simulink model "F4PhantomModelV3"  (R2023b)
settings: Solver=VariableStepAuto  StartTime=0.0  StopTime=10.0  RelTol=1e-3
values from neighbouring files (symbols this model uses):
  FTx = 0    [F4ModelCode.m]    (also in F4ModelCodeV2.m; F4ModelCodeV2Q2PartD.m)
  fTx = 0    [F4ModelCode.m]    (also in F4ModelCodeV2.m; F4ModelCodeV2Q2PartD.m)
  FTy = 0    [F4ModelCode.m]    (also in F4ModelCodeV2.m; F4ModelCodeV2Q2PartD.m)
  fTy = 0    [F4ModelCode.m]    (also in F4ModelCodeV2.m; F4ModelCodeV2Q2PartD.m)
  FTz = 0    [F4ModelCode.m]    (also in F4ModelCodeV2.m; F4ModelCodeV2Q2PartD.m)
  fTz = 0    [F4ModelCode.m]    (also in F4ModelCodeV2.m; F4ModelCodeV2Q2PartD.m)
  g = -32.2    [F4ModelCode.m]    (also in F4ModelCodeV2.m; F4ModelCodeV2Q2PartD.m; F4PhantomModelCode.m)
  Hw3Coeffs = [c_L_alpha c_L_delta_E c_L_i_H c_m_alpha c_m_delta_E c_m_i_H c_L_alphadot c_L_q c_m_alphadot c_m_q c_D_alpha]    [F4ModelCode.m]    (also in F4ModelCodeV2.m; F4ModelCodeV2Q2PartD.m; F4PhantomModelCode.m = [c_L_alpha c_L_delta_E c_L_i_H c_m_alpha c_m_delta_E c_m_i_H)
  Hw4Coeffs = [c_Y_beta c_Y_delta_A c_Y_delta_R c_n_beta c_n_delta_A c_n_delta_R c_l_beta c_l_delta_A c_l_delta_R c_l_p c_Y_p c_n_p c_l_r c_Y_r c_n_r]    [F4ModelCode.m]    (also in F4ModelCodeV2.m; F4ModelCodeV2Q2PartD.m; F4PhantomModelCode.m)
  InitialInputs = [qbar1 S_ft2 c_D_1 c_L_1 cbar_ft c_m_1 uv b_ft alphadot]    [F4ModelCode.m]    (also in F4ModelCodeV2.m; F4ModelCodeV2Q2PartD.m)
  LT = 0    [F4ModelCode.m]    (also in F4ModelCodeV2Q2PartD.m)
  lT = 0    [F4ModelCode.m]    (also in F4ModelCodeV2Q2PartD.m)
  mass = Weight/32.2    (= 1211.18012422)    [F4ModelCode.m]    (also in F4ModelCodeV2.m; F4ModelCodeV2Q2PartD.m; F4PhantomModelCode.m = 1212.157)
  MT = 0    [F4ModelCode.m]    (also in F4ModelCodeV2Q2PartD.m)
  mT = 0    [F4ModelCode.m]    (also in F4ModelCodeV2Q2PartD.m)
  NT = 0    [F4ModelCode.m]    (also in F4ModelCodeV2Q2PartD.m)
  nT = 0    [F4ModelCode.m]    (also in F4ModelCodeV2Q2PartD.m)
  P1 = 0    [F4ModelCode.m]    (also in F4ModelCodeV2.m; F4ModelCodeV2Q2PartD.m; F4PhantomModelCode.m)
  q0 = angle2quat(phidot,thetadot,psidot)    [F4ModelCode.m]    (also in F4ModelCodeV2.m; F4ModelCodeV2Q2PartD.m)
  U1 = V_P_1 * cos(alpha_rad)    [F4ModelCode.m]    (also in F4ModelCodeV2.m; F4ModelCodeV2Q2PartD.m)
  uCoeffs = [c_L_u c_D_u c_m_u]    [F4ModelCode.m]    (also in F4ModelCodeV2.m; F4ModelCodeV2Q2PartD.m; F4PhantomModelCode.m = [c_L_u c_D_u])
  uk = [c_D_delta_E c_D_q c_D_i_H c_Y_1 c_Y_betadot c_l_betadot c_n_1 c_n_betadot]    [F4ModelCode.m]    (also in F4ModelCodeV2.m; F4ModelCodeV2Q2PartD.m)
  V_P_1 = 875.6    [F4ModelCode.m]    (also in F4ModelCodeV2.m; F4ModelCodeV2Q2PartD.m; F4PhantomModelCode.m = 0)
  W1 = V_P_1 * sin(alpha_rad)    [F4ModelCode.m]    (also in F4ModelCodeV2.m; F4ModelCodeV2Q2PartD.m)
undefined symbols (not defined in the file or in its folder): THETA1
settings Model: Creator=Owner  LastModifiedBy=Owner

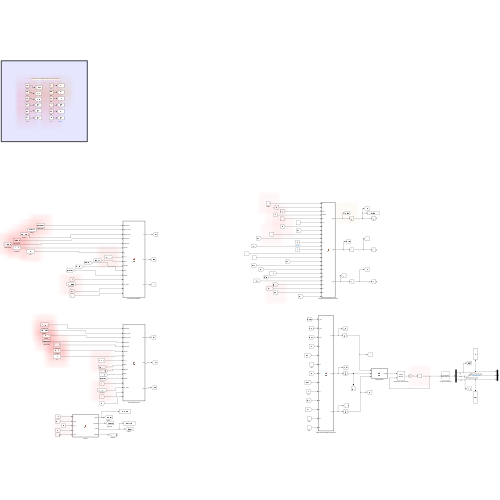
[thumbnail: Simulink's stored preview of the top-level diagram]
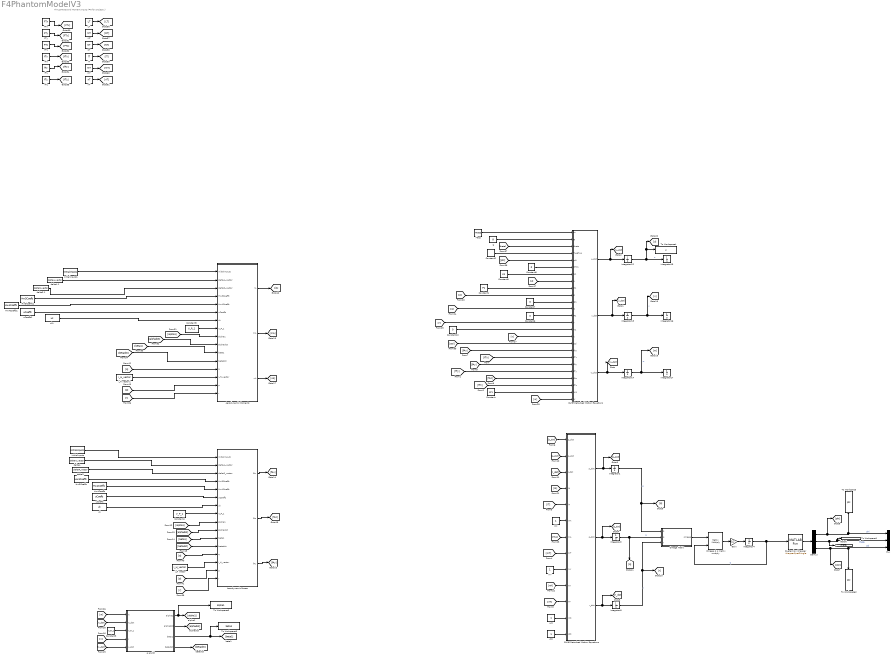
== system F4PhantomModelV3 ==
  note: Thrust Force and Moment Inputs (=0 for project 1)
  Aerodynamic Forces : MATLAB Function  TreatAsAtomicUnit=on
  Aerodynamic Moments : MATLAB Function  TreatAsAtomicUnit=on
  CAME Perturbed Motion Equations : MATLAB Function  TreatAsAtomicUnit=on
  CLME Perturbed Motion Equations : MATLAB Function  TreatAsAtomicUnit=on
  Constant : Constant  Value=W1
  Constant1 : Constant  Value=P1
  Constant{6..8,10} (4 alike) : Constant  Value=0
  Constant2 : Constant  Value=THETA1
  Constant3 : Constant  Value=V_P_1
  Constant4 : Constant  Value=V_P_1
  Constant5 : Constant  Value=V_P_1
  Constant9 : Constant  Value=U1
  Demux : Demux  Outputs=3
  FTx : Constant  Value=FTx
  FTy : Constant  Value=FTy
  FTz : Constant  Value=FTz
  Gain : Gain  Gain=1/2
  Hw3Coeffs : Constant  Value=Hw3Coeffs
  Hw3Coeffs1 : Constant  Value=Hw3Coeffs
  Hw4Coeffs : Constant  Value=Hw4Coeffs
  Hw4Coeffs1 : Constant  Value=Hw4Coeffs
  "IXX " : Constant
  IXZ : Constant
  IYY : Constant
  IZZ : Constant
  InitialInputs : Constant  Value=InitialInputs
  InitialInputs1 : Constant  Value=InitialInputs
  Integrator{1..3,12..17} (9 alike) : Integrator
  Integrator4 : Integrator  InitialCondition=q0
  LT : Constant  Value=LT
  MT : Constant  Value=MT
  Mass : Constant  Value=mass
  Mux : Mux  Inputs=3
  NT : Constant  Value=NT
  Omega & q matrix mutiply : Product  Multiplication=Matrix(*)
  Omega Matrix : MATLAB Function  TreatAsAtomicUnit=on
  Quaternion Wrapper : MATLABFcn  MATLABFcn=WrapperQuat2Angle
  To Workspace : ToWorkspace  VariableName=phi  SaveFormat=Timeseries  SampleTime=-1
  To Workspace1 : ToWorkspace  VariableName=theta  SaveFormat=Timeseries  SampleTime=-1
  To Workspace2 : ToWorkspace  VariableName=psi  SaveFormat=Timeseries  SampleTime=-1
  To Workspace3 : ToWorkspace  VariableName=beta1  SampleTime=-1
      settings: Save2DSignal=2-D array (concatenate along first dimension)
  To Workspace4 : ToWorkspace  VariableName=u  SaveFormat=Timeseries  SampleTime=-1
  To Workspace6 : ToWorkspace  VariableName=alpha1  SaveFormat=Timeseries  SampleTime=-1
  "deltaA " : FromWorkspace  VariableName=deltaA_vector  OutDataTypeStr=double
  deltaA 1 : FromWorkspace  VariableName=deltaA_vector  OutDataTypeStr=double
  "deltaR " : FromWorkspace  VariableName=deltaR_vector  OutDataTypeStr=double
  deltaR 1 : FromWorkspace  VariableName=deltaR_vector  OutDataTypeStr=double
  fTx : Constant  Value=fTx
  fTy : Constant  Value=fTy
  fTz : Constant  Value=fTz
  g : Constant  Value=g
  "i_H vector " : FromWorkspace  VariableName=i_H_vector
  i_H vector 1 : FromWorkspace  VariableName=i_H_vector
  lT : Constant  Value=lT
  mT : Constant  Value=mT
  nT : Constant  Value=nT
  uCoeffs : Constant  Value=uCoeffs
  uCoeffs1 : Constant  Value=uCoeffs
  uk : Constant  Value=uk
  uk1 : Constant  Value=uk
  α and β : MATLAB Function  TreatAsAtomicUnit=on
  wires:
  CAME Perturbed Motion Equations/2(q_dot) -> [q_dot], Integrator2/1
  CAME Perturbed Motion Equations/3(r_dot) -> [r_dot], Integrator3/1
  CAME Perturbed Motion Equations/1(p_dot) -> [p_dot], Integrator1/1
  IZZ/1 -> CAME Perturbed Motion Equations/13(IZZ)
  [nA] -> CAME Perturbed Motion Equations/10(nA)
  [lA] -> CAME Perturbed Motion Equations/4(lA)
  "IXX "/1 -> CAME Perturbed Motion Equations/6(IXX)
  [mA] -> CAME Perturbed Motion Equations/7(mA)
  IYY/1 -> CAME Perturbed Motion Equations/9(IYY)
  IXZ/1 -> CAME Perturbed Motion Equations/12(IXZ)
  FTx/1 -> [FTx]
  fTz/1 -> [fTz]
  fTy/1 -> [fTy]
  nT/1 -> [nT]
  mT/1 -> [mT]
  LT/1 -> [LT]
  lT/1 -> [lT]
  NT/1 -> [NT]
  FTz/1 -> [FTz]
  MT/1 -> [MT]
  FTy/1 -> [FTy]
  fTx/1 -> [fTx]
  Mass/1 -> CLME Perturbed Motion Equations/1(m)
  [fAx] -> CLME Perturbed Motion Equations/18(fAx)
  CLME Perturbed Motion Equations/1(u_dot) -> [u_dot], Integrator12/1
  [psi] -> CLME Perturbed Motion Equations/17(psi)
  [q] -> CLME Perturbed Motion Equations/12(q)
  g/1 -> CLME Perturbed Motion Equations/2(g)
  Integrator13/1 -> [v], Integrator16/1  "v"
  Constant9/1 -> CLME Perturbed Motion Equations/7(U1)
  CLME Perturbed Motion Equations/3(w_dot) -> Integrator14/1, [w_dot]
  CLME Perturbed Motion Equations/2(v_dot) -> [v_dot], Integrator13/1
  [p] -> CLME Perturbed Motion Equations/10(p)
  Constant10/1 -> CLME Perturbed Motion Equations/15(V1)
  [phi] -> CLME Perturbed Motion Equations/5(phi)
  [r] -> CLME Perturbed Motion Equations/14(r)
  Integrator12/1 -> [u], To Workspace4/1, Integrator15/1  "u"
  [fAy] -> CLME Perturbed Motion Equations/20(fAy)
  [fAz] -> CLME Perturbed Motion Equations/22(fAz)
  [theta] -> CLME Perturbed Motion Equations/3(theta)
  Integrator14/1 -> Integrator17/1, [w]  "w"
  [fTx] -> CLME Perturbed Motion Equations/19(fTx)
  [fTy] -> CLME Perturbed Motion Equations/21(fTy)
  [fTz] -> CLME Perturbed Motion Equations/23(fTz)
  Constant/1 -> CLME Perturbed Motion Equations/24(W1)
  Constant1/1 -> CLME Perturbed Motion Equations/9(P1)
  Constant2/1 -> CLME Perturbed Motion Equations/4(THETA1)
  [nT] -> CAME Perturbed Motion Equations/11(nT)
  [mT] -> CAME Perturbed Motion Equations/8(mT)
  [lT] -> CAME Perturbed Motion Equations/5(lT)
  Integrator1/1 -> Omega Matrix/1(p), [p]  "p"
  [p_dot] -> CAME Perturbed Motion Equations/1("p_dot ")
  [q_dot] -> CAME Perturbed Motion Equations/2("q_dot ")
  [r_dot] -> CAME Perturbed Motion Equations/3("r_dot ")
  Integrator2/1 -> Omega Matrix/2(q), [q]  "q"
  Integrator3/1 -> [r], Omega Matrix/3(r)  "r"
  Gain/1 -> Integrator4/1
  Omega & q matrix mutiply/1 -> Gain/1
  Omega Matrix/1(omega) -> Omega & q matrix mutiply/1
  Integrator4/1 -> Quaternion Wrapper/1, Omega & q matrix mutiply/2  "q"
  Quaternion Wrapper/1 -> Demux/1
  Demux/1 -> Mux/1, To Workspace/1, [phi]  "phi"
  Demux/2 -> Mux/2, To Workspace1/1, [theta]  "theta"
  Demux/3 -> Mux/3, To Workspace2/1, [psi]  "psi"
  [r] -> Aerodynamic Forces/16(r)
  [alpha1] -> Aerodynamic Forces/9(alpha1)
  [v_dot] -> α and β/5(v_dot)
  "i_H vector "/1 -> Aerodynamic Forces/14(i_H_vector)
  uCoeffs/1 -> Aerodynamic Forces/6(uCoeffs)
  [w_dot] -> α and β/2(w_dot)
  [beta1] -> Aerodynamic Forces/11(beta1)
  [q] -> Aerodynamic Forces/13(q)
  InitialInputs/1 -> Aerodynamic Forces/1(InitialInputs)
  uk/1 -> Aerodynamic Forces/7(uk)
  Hw4Coeffs/1 -> Aerodynamic Forces/5(Hw4Coeffs)
  α and β/3(beta1) -> [beta1], To Workspace3/1
  Aerodynamic Forces/3(fAy) -> [fAy]
  Constant5/1 -> Aerodynamic Moments/8(V_P_1)
  Aerodynamic Moments/3(nA) -> [nA]
  Hw3Coeffs/1 -> Aerodynamic Forces/4(Hw3Coeffs)
  Constant4/1 -> Aerodynamic Forces/8(V_P_1)
  α and β/1(alpha1) -> To Workspace6/1, [alpha1]
  Aerodynamic Moments/1(lA) -> [lA]
  Constant3/1 -> α and β/3(V_P_1)
  [alphadot] -> Aerodynamic Forces/10(alphadot)
  "deltaA "/1 -> Aerodynamic Forces/2(deltaA_vector)
  [w] -> α and β/1(w)
  α and β/2(alphadot) -> [alphadot]
  [v] -> α and β/4(v)
  "deltaR "/1 -> Aerodynamic Forces/3(deltaR_vector)
  α and β/4(betadot) -> [betadot]
  Aerodynamic Forces/2(fAz) -> [fAz]
  Aerodynamic Moments/2(mA) -> [mA]
  Aerodynamic Forces/1(fAx) -> [fAx]
  [betadot] -> Aerodynamic Forces/12(betadot)
  [p] -> Aerodynamic Forces/15(p)
  [u] -> CLME Perturbed Motion Equations/8(u)
  [v] -> CLME Perturbed Motion Equations/16(v)
  [w] -> CLME Perturbed Motion Equations/25(w)
  deltaA 1/1 -> Aerodynamic Moments/2(deltaA_vector)
  Hw4Coeffs1/1 -> Aerodynamic Moments/5(Hw4Coeffs)
  Hw3Coeffs1/1 -> Aerodynamic Moments/4(Hw3Coeffs)
  uCoeffs1/1 -> Aerodynamic Moments/6(uCoeffs)
  deltaR 1/1 -> Aerodynamic Moments/3(deltaR_vector)
  uk1/1 -> Aerodynamic Moments/7(uk)
  InitialInputs1/1 -> Aerodynamic Moments/1(InitialInputs)
  [alpha1] -> Aerodynamic Moments/9(alpha1)
  [alphadot] -> Aerodynamic Moments/10(alphadot)
  [beta1] -> Aerodynamic Moments/11(beta1)
  [betadot] -> Aerodynamic Moments/12(betadot)
  [q] -> Aerodynamic Moments/13(q)
  i_H vector 1/1 -> Aerodynamic Moments/14(i_H_vector)
  [p] -> Aerodynamic Moments/15(p)
  [r] -> Aerodynamic Moments/16(r)
  Constant6/1 -> CLME Perturbed Motion Equations/13(R1)
  Constant7/1 -> CLME Perturbed Motion Equations/11(Q1)
  Constant8/1 -> CLME Perturbed Motion Equations/6(PHI1)

== matlab function F4PhantomModelV3/CLME Perturbed Motion Equations ==
  data: m input; u_dot output; g input; theta input; THETA1 input; phi input; PHI1 input; U1 input; u input; P1 input; p input; Q1 input; q input; R1 input; r input; v_dot output; w_dot output; V1 input; v input; psi input; fAx input; fTx input; fAy input; fTy input; fAz input; fTz input; W1 input; w input
function [u_dot, v_dot, w_dot] = fcn(m, g, theta, THETA1, phi, PHI1, U1, u, P1, p, Q1, q, R1, r, V1, v, psi, fAx, fTx, fAy, fTy, fAz, fTz, W1, w)



%u_dot = (1/m) * ((-m*g*theta*cosd(THETA1)) + (fAx + fTx) - (Q1*w) - (q*W1) + (R1*v) + (r*V1));
%v_dot = (1/m) * (((-m*g*theta*sind(PHI1)*sind(THETA1))+(m*g*phi*cosd(PHI1)*cosd(THETA1))) + (fAy + fTy) - (U1*r) - (u*R1) + (P1*w) + (p*W1));
%w_dot = (1/m) * (((-m*g*theta*cosd(PHI1)*sind(THETA1))-(m*g*phi*sind(PHI1)*cosd(THETA1))) + (fAz + fTz) - (P1*v) - (V1*p) + (Q1*u) + (U1*q));

u_dot = (1/m) * ((-m*g*theta*cosd(THETA1)) + (fAx + fTx) - (q*W1));
v_dot = (1/m) * ((m*g*phi*cosd(THETA1)) + (fAy+fTy) - (U1*r) + (p*W1));
w_dot = (1/m) * ((-m*g*theta*sind(THETA1)) + (fAz + fTz) + (U1*q));

== matlab function F4PhantomModelV3/CAME Perturbed Motion Equations ==
  data: p_dot input; p_dot output; q_dot input; r_dot input; lA input; lT input; IXX input; mA input; mT input; IYY input; nA input; nT input; IXZ input; IZZ input; q_dot output; r_dot output
function [p_dot, q_dot, r_dot] = fcn(p_dot, q_dot, r_dot, lA, lT, IXX, mA, mT, IYY, nA, nT, IXZ, IZZ)
%CAME - Still Needs to be fixed
%P_dot = ((la+lt)+(R_dot.*IXZ)+(P.*Q.*IXZ)-((R*Q).*(IZZ-IYY)))./(IXX);
%Q_dot = ((ma+mt)-(R_dot.*IXZ)+(P.*Q.*IXZ)-(R*Q).*(IZZ-IYY))./(IYY);
%R_dot = ((nA+nT) + (P_dot*IXZ) - (((P1*q)+(p*Q1))*(IYY-IXX)) - (((Q1*r)+(R1*q))*IXZ))/(IZZ);

p_dot = ((r_dot*IXZ) + (lA+lT))/IXX;
q_dot = (mA+mT)/IYY;
r_dot = ((nA+nT) + (p_dot*IXZ))/IZZ;

%Need to reorganzie to solve for it

== matlab function F4PhantomModelV3/Aerodynamic Forces ==
  data: InitialInputs input; deltaA_vector input; deltaR_vector input; Hw3Coeffs input; Hw4Coeffs input; uCoeffs input; uk input; V_P_1 input; alpha1 input; alphadot input; beta1 input; betadot input; q input; i_H_vector input; fAx output; fAz output; fAy output; p input; r input
function [ fAx, fAz,  fAy]  = fcn(InitialInputs, deltaA_vector, deltaR_vector, Hw3Coeffs, Hw4Coeffs, uCoeffs, uk, V_P_1, alpha1, alphadot, beta1, betadot, q, i_H_vector, p, r)
qbar1 = InitialInputs(1); S_ft2 = InitialInputs(2); c_D_1 = InitialInputs(3); c_L_1 = InitialInputs(4); cbar_ft = InitialInputs(5); c_m_1 = InitialInputs(6); uv = InitialInputs(7); b_ft = InitialInputs(8);
% deltaA_vector = CSv(1); deltaR_vector = CSv(2); deltaS_vector = CSv(3); 
% deltaA = CSc(1); deltaS = CSc(2); deltaR = CSc(3);
c_L_alpha = Hw3Coeffs(1); c_L_delta_E = Hw3Coeffs(2); c_L_i_H = Hw3Coeffs(3); c_m_alpha = Hw3Coeffs(4); c_m_delta_E = Hw3Coeffs(5); c_m_i_H = Hw3Coeffs(6); c_L_alphadot = Hw3Coeffs(7); c_L_q = Hw3Coeffs(8); c_m_alphadot = Hw3Coeffs(9); c_m_q = Hw3Coeffs(10); c_D_alpha = Hw3Coeffs(11);
c_Y_beta = Hw4Coeffs(1); c_Y_delta_A = Hw4Coeffs(2); c_Y_delta_R = Hw4Coeffs(3); c_n_beta = Hw4Coeffs(4); c_n_delta_A = Hw4Coeffs(5); c_n_delta_R = Hw4Coeffs(6); c_l_beta = Hw4Coeffs(7); c_l_delta_A = Hw4Coeffs(8); c_l_delta_R = Hw4Coeffs(9); c_l_p = Hw4Coeffs(10); c_Y_p = Hw4Coeffs(11); c_n_p = Hw4Coeffs(12); c_l_r = Hw4Coeffs(13); c_Y_r = Hw4Coeffs(14); c_n_r = Hw4Coeffs(15);
c_L_u = uCoeffs(1); c_D_u = uCoeffs(2); c_m_u = uCoeffs(3); 
c_D_delta_E = uk(1);  c_D_q = uk(2); c_D_i_H = uk(3); c_Y_1 = uk(4); c_Y_betadot = uk(5); c_l_betadot = uk(6); c_n_1 = uk(7); c_n_betadot = uk(8);

deltaE = 0;

%FAx = -qbar1*S_ft2*c_D_1;
fAx = (qbar1*S_ft2)*(((-(c_D_u+(2*c_D_1)))*(uv/V_P_1)) + ((c_D_alpha + c_L_1)*(alpha1)) - c_D_alpha*((alphadot*cbar_ft)/(2*V_P_1)) - c_D_q*((q*cbar_ft)/(2*V_P_1)) - (c_D_delta_E*deltaE)-(c_D_i_H*i_H_vector));

%FAz = -qbar1*S_ft2*c_L_1;
fAz = (qbar1*S_ft2)*(((-(c_L_u+(2*c_L_1)))*(uv/V_P_1)) + ((c_L_alpha + c_D_1)*(alpha1)) - c_L_alphadot*((alphadot*cbar_ft)/(2*V_P_1)) - c_L_q*((q*cbar_ft)/(2*V_P_1)) - (c_L_delta_E*deltaE)-(c_L_i_H*i_H_vector));

%FAy = -qbar1*S_ft2*c_Y_1;
fAy = -qbar1*S_ft2 * ((c_Y_beta*beta1) + c_Y_betadot * ((betadot*b_ft)/(2*V_P_1)) + c_Y_p*((p*b_ft)/(2*V_P_1)) + c_Y_r * ((r*b_ft)/(2*V_P_1)) +(c_Y_delta_A * deltaA_vector) + (c_Y_delta_R*deltaR_vector));

%LA = -qbar1*S_ft2*b_ft*c_L_1;
% lA = -qbar1*S_ft2*b_ft*((c_l_beta*beta1) + c_l_betadot * ((betadot*b_ft)/(2*V_P_1)) + c_l_p*((p*b_ft)/(2*V_P_1)) + c_l_r * ((r*b_ft)/(2*V_P_1)) +(c_l_delta_A * deltaA_vector) + (c_l_delta_R*deltaR_vector));
% 
% %MA = -qbar1*S_ft2*cbar_ft*c_m_1; %%%%This line is throwing an error
% mA = (qbar1*S_ft2*cbar_ft)*(((-(c_m_u+(2*c_m_1)))*(uv/V_P_1)) + (c_m_alpha*alpha1) + c_m_alphadot*((alphadot*cbar_ft)/(2*V_P_1)) + c_m_q*((q*cbar_ft)/(2*V_P_1)) + (c_m_delta_E*deltaE)+(c_L_i_H*i_H_vector));
% 
% %NA = -qbar1*S_ft2*b_ft*c_n_1;
% nA = -qbar1*S_ft2*b_ft*((c_n_beta*beta1) + c_n_betadot * ((betadot*b_ft)/(2*V_P_1)) + c_n_p*((p*b_ft)/(2*V_P_1)) + c_n_r * ((r*b_ft)/(2*V_P_1)) +(c_n_delta_A * deltaA_vector) + (c_n_delta_R*deltaR_vector));

%Need to get rid of fAy and lA and nA, leave MA and mA

== matlab function F4PhantomModelV3/Omega Matrix ==
  data: p input; omega output; q input; r input
function omega = fcn(p,q,r)


wx = p;
wy = q;
wz = r;
omega = [0 -wx -wy -wz;
         wx 0 wz -wy;
         wy -wz 0 wx;
         wz wy -wx 0];

== matlab function F4PhantomModelV3/Aerodynamic Moments ==
  data: InitialInputs input; deltaA_vector input; deltaR_vector input; Hw3Coeffs input; Hw4Coeffs input; uCoeffs input; uk input; V_P_1 input; alpha1 input; alphadot input; beta1 input; betadot input; q input; i_H_vector input; lA output; mA output; nA output; p input; r input
function [lA,  mA, nA]  = fcn(InitialInputs, deltaA_vector, deltaR_vector, Hw3Coeffs, Hw4Coeffs, uCoeffs, uk, V_P_1, alpha1, alphadot, beta1, betadot, q, i_H_vector, p, r)
qbar1 = InitialInputs(1); S_ft2 = InitialInputs(2); c_D_1 = InitialInputs(3); c_L_1 = InitialInputs(4); cbar_ft = InitialInputs(5); c_m_1 = InitialInputs(6); uv = InitialInputs(7); b_ft = InitialInputs(8);
% deltaA_vector = CSv(1); deltaR_vector = CSv(2); deltaS_vector = CSv(3); 
% deltaA = CSc(1); deltaS = CSc(2); deltaR = CSc(3);
c_L_alpha = Hw3Coeffs(1); c_L_delta_E = Hw3Coeffs(2); c_L_i_H = Hw3Coeffs(3); c_m_alpha = Hw3Coeffs(4); c_m_delta_E = Hw3Coeffs(5); c_m_i_H = Hw3Coeffs(6); c_L_alphadot = Hw3Coeffs(7); c_L_q = Hw3Coeffs(8); c_m_alphadot = Hw3Coeffs(9); c_m_q = Hw3Coeffs(10); c_D_alpha = Hw3Coeffs(11);
c_Y_beta = Hw4Coeffs(1); c_Y_delta_A = Hw4Coeffs(2); c_Y_delta_R = Hw4Coeffs(3); c_n_beta = Hw4Coeffs(4); c_n_delta_A = Hw4Coeffs(5); c_n_delta_R = Hw4Coeffs(6); c_l_beta = Hw4Coeffs(7); c_l_delta_A = Hw4Coeffs(8); c_l_delta_R = Hw4Coeffs(9); c_l_p = Hw4Coeffs(10); c_Y_p = Hw4Coeffs(11); c_n_p = Hw4Coeffs(12); c_l_r = Hw4Coeffs(13); c_Y_r = Hw4Coeffs(14); c_n_r = Hw4Coeffs(15);
c_L_u = uCoeffs(1); c_D_u = uCoeffs(2); c_m_u = uCoeffs(3); 
c_D_delta_E = uk(1);  c_D_q = uk(2); c_D_i_H = uk(3); c_Y_1 = uk(4); c_Y_betadot = uk(5); c_l_betadot = uk(6); c_n_1 = uk(7); c_n_betadot = uk(8);

deltaE = 0;

% %FAx = -qbar1*S_ft2*c_D_1;
% fAx = (qbar1*S_ft2)*(((-(c_D_u+(2*c_D_1)))*(uv/V_P_1)) + ((c_D_alpha + c_L_1)*(alpha1)) - c_D_alpha*((alphadot*cbar_ft)/(2*V_P_1)) - c_D_q*((q*cbar_ft)/(2*V_P_1)) - (c_D_delta_E*deltaE)-(c_D_i_H*i_H_vector));
% 
% %FAz = -qbar1*S_ft2*c_L_1;
% fAz = (qbar1*S_ft2)*(((-(c_L_u+(2*c_L_1)))*(uv/V_P_1)) + ((c_L_alpha + c_D_1)*(alpha1)) - c_L_alphadot*((alphadot*cbar_ft)/(2*V_P_1)) - c_L_q*((q*cbar_ft)/(2*V_P_1)) - (c_L_delta_E*deltaE)-(c_L_i_H*i_H_vector));
% 
% %FAy = -qbar1*S_ft2*c_Y_1;
% fAy = -qbar1*S_ft2 * ((c_Y_beta*beta1) + c_Y_betadot * ((betadot*b_ft)/(2*V_P_1)) + c_Y_p*((p*b_ft)/(2*V_P_1)) + c_Y_r * ((r*b_ft)/(2*V_P_1)) +(c_Y_delta_A * deltaA_vector) + (c_Y_delta_R*deltaR_vector));

%LA = -qbar1*S_ft2*b_ft*c_L_1;
lA = -qbar1*S_ft2*b_ft*((c_l_beta*beta1) + c_l_betadot * ((betadot*b_ft)/(2*V_P_1)) + c_l_p*((p*b_ft)/(2*V_P_1)) + c_l_r * ((r*b_ft)/(2*V_P_1)) +(c_l_delta_A * deltaA_vector) + (c_l_delta_R*deltaR_vector));
% 
% %MA = -qbar1*S_ft2*cbar_ft*c_m_1; %%%%This line is throwing an error
mA = (qbar1*S_ft2*cbar_ft)*(((-(c_m_u+(2*c_m_1)))*(uv/V_P_1)) + (c_m_alpha*alpha1) + c_m_alphadot*((alphadot*cbar_ft)/(2*V_P_1)) + c_m_q*((q*cbar_ft)/(2*V_P_1)) + (c_m_delta_E*deltaE)+(c_L_i_H*i_H_vector));
% 
% %NA = -qbar1*S_ft2*b_ft*c_n_1;
nA = -qbar1*S_ft2*b_ft*((c_n_beta*beta1) + c_n_betadot * ((betadot*b_ft)/(2*V_P_1)) + c_n_p*((p*b_ft)/(2*V_P_1)) + c_n_r * ((r*b_ft)/(2*V_P_1)) +(c_n_delta_A * deltaA_vector) + (c_n_delta_R*deltaR_vector));

%Need to get rid of fAy and lA and nA, leave MA and mA

== matlab function F4PhantomModelV3/α and β ==
  data: w input; alpha1 output; alphadot output; beta1 output; w_dot input; V_P_1 input; v input; v_dot input; betadot output
function [alpha1, alphadot, beta1, betadot] = fcn(w, w_dot, V_P_1, v, v_dot)

alpha1 = w/V_P_1;

alphadot = w_dot/V_P_1;

beta1 = v/V_P_1;

betadot = v_dot/V_P_1;
